simulink model "LQ_simulation"  (R2024b)
settings: Solver=VariableStepAuto  StartTime=0.0  StopTime=10.0  RelTol=1e-3
values from neighbouring files (symbols this model uses):
  A_kf = A_ext - L_kf*C_meas    [SS_model_LQ.m]
  A_x = [0, 1 ... (first row only)    [SS_model_LQ.m]
  B_kf = [L_kf B_ext]    [SS_model_LQ.m]
  B_x = [0; k2]    [SS_model_LQ.m]
  C_kf = eye(3)    [SS_model_LQ.m]
  C_x = [1, 0]    [SS_model_LQ.m]
  D_kf = zeros(3,3)    [SS_model_LQ.m]
  D_x = 0    [SS_model_LQ.m]
  K_lq = lqr(A_ext, B_ext, Q_lq, R_lq)    [SS_model_LQ.m]
  K_ref = -1/(C_pos_ext*((A_ext - B_ext*K_lq)\B_ext))    [SS_model_LQ.m]
  Kg = 3    [LQI_Giuse_code.m]    (also in SS_model_LQ.m)
  Ki_i = Ki_p/Ti    [LQI_Giuse_code.m]    (also in SS_model_LQ.m = 1650.02619)
  Kp_i = 72.795273    [SS_model_LQ.m]
  x_e = [x1_e, x2_e]    [LQI_Giuse_code.m]    (also in SS_model_LQ.m = 0.007)
undefined symbols (not defined in the file or in its folder): G_i_den, G_i_num
libraries: slpidlib x1
settings Model: Creator=edoardo  LastModifiedBy=edoardo

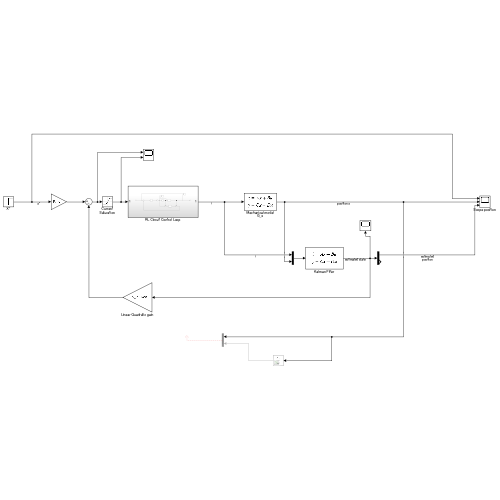
[thumbnail: Simulink's stored preview of the top-level diagram]
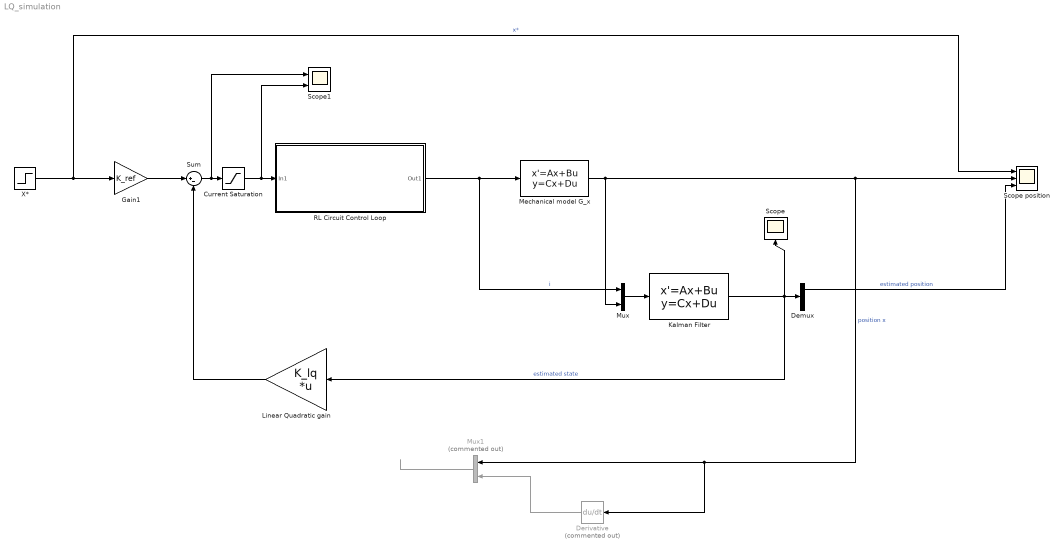
== system LQ_simulation ==
  Current Saturation : Saturate  UpperLimit=3  LowerLimit=-3
  Demux : Demux  Outputs=2
  Derivative : Derivative  Commented=on
  Gain1 : Gain  Gain=K_ref
  Kalman Filter : StateSpace  A=A_kf  B=B_kf  C=C_kf  D=D_kf  InitialCondition=0
  Linear Quadratic gain : Gain  Gain=K_lq  Multiplication=Matrix(K*u) (u vector)
  Mechanical model G_x : StateSpace  A=A_x  B=B_x  C=C_x  D=D_x  InitialCondition=0
  Mux : Mux  Inputs=2
  Mux1 : Mux  Commented=on  Inputs=2
  RL Circuit Control Loop : Subsystem
  Scope : Scope
  Scope position : Scope  NumInputPorts=3
  Scope1 : Scope  NumInputPorts=2
  Sum : Sum  Inputs=|+-
  X* : Step  After=x_e  SampleTime=0
  wires:
  RL Circuit Control Loop/1(Out1) -> Mux/1, Mechanical model G_x/1  "i"
  X*/1 -> Gain1/1, Scope position/1  "x*"
  Mechanical model G_x/1 -> Mux/2, Scope position/2, Mux1/1, Derivative/1  "position x"
  Mux/1 -> Kalman Filter/1
  Kalman Filter/1 -> Linear Quadratic gain/1, Scope/1, Demux/1  "estimated state"
  Linear Quadratic gain/1 -> Sum/2
  Sum/1 -> Scope1/1, Current Saturation/1
  Demux/1 -> Scope position/3  "estimated position"
  Current Saturation/1 -> Scope1/2, RL Circuit Control Loop/1(In1)
  Gain1/1 -> Sum/1
  Mux1/1 -> ?
  Derivative/1 -> Mux1/2

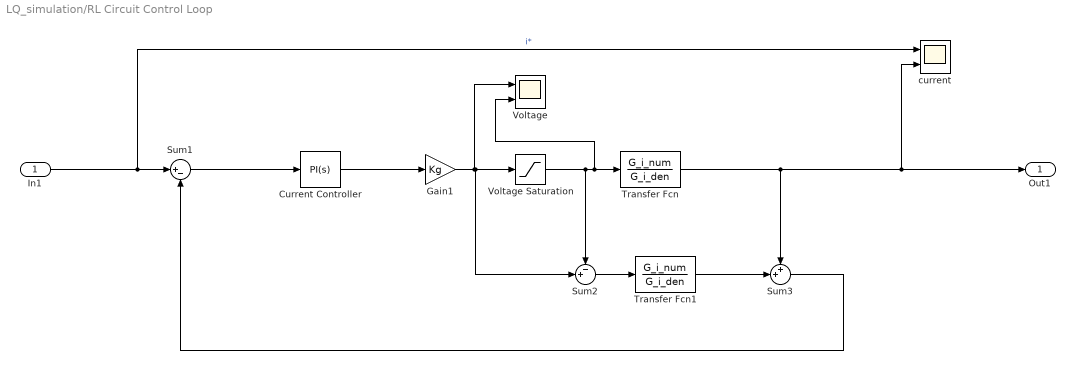
== system LQ_simulation/RL Circuit Control Loop ==
  In1 : Inport
  Current Controller : slpidlib/PID Controller  Controller=PI  Form=Parallel  TimeDomain=Continuous-time  UseExternalTs=off  SampleTime=-1  IntegratorMethod=Forward Euler  FilterMethod=Forward Euler  ControllerParametersSource=internal  P=Kp_i  I=Ki_i  UseKiTs=off  D=0  UseExternalDerivativeSource=off  N=100  UseFilter=on  TunerSelectOption=Transfer Function Based (PID Tuner App)  InitialConditionSource=internal  InitialConditionForIntegrator=0  InitialConditionForFilter=0  DifferentiatorICPrevScaledInput=0  ExternalReset=none  TrackingMode=off  Kt=1  LimitOutput=off  SatLimitsSource=internal  UpperSaturationLimit=inf  LowerSaturationLimit=-inf  LinearizeAsGain=on  AntiWindupMode=none  Kb=1  LimitIntegrator=off  UpperIntegratorSaturationLimit=inf  LowerIntegratorSaturationLimit=-inf  POutMin=[]  POutMax=[]  IOutMin=[]  IOutMax=[]  DOutMin=[]  DOutMax=[]  NOutMin=[]  NOutMax=[]  SumOutMin=[]  SumOutMax=[]  SaturationOutMin=[]  SaturationOutMax=[]  PParamMin=[]  PParamMax=[]  IParamMin=[]  IParamMax=[]  DParamMin=[]  DParamMax=[]  NParamMin=[]  NParamMax=[]  KbParamMin=[]  KbParamMax=[]  KtParamMin=[]  KtParamMax=[]  KbOutMin=[]  KbOutMax=[]  KtOutMin=[]  KtOutMax=[]  IntegratorOutMin=[]  IntegratorOutMax=[]  FilterOutMin=[]  FilterOutMax=[]  SumI1OutMin=[]  SumI1OutMax=[]  SumI2OutMin=[]  SumI2OutMax=[]  SumI3OutMin=[]  SumI3OutMax=[]  SumI4OutMin=[]  SumI4OutMax=[]  SumDOutMin=[]  SumDOutMax=[]  DifferentiatorOutMin=[]  DifferentiatorOutMax=[]  FilterDiffOutCoefMin=[]  FilterDiffOutCoefMax=[]  ReciprocalOutMin=[]  ReciprocalOutMax=[]  SumDenOutMin=[]  SumDenOutMax=[]  SumNumOutMin=[]  SumNumOutMax=[]  DivideOutMin=[]  DivideOutMax=[]  UdiffTsProdOutMin=[]  UdiffTsProdOutMax=[]  NTsProdOutMin=[]  NTsProdOutMax=[]  UintegralTsProdOutMin=[]  UintegralTsProdOutMax=[]  UngainTsProdOutMin=[]  UngainTsProdOutMax=[]  ClampingZeroOutDataTypeStr=Inherit: Inherit via back propagation  ClampingZeroOutMin=[]  ClampingZeroOutMax=[]  FilterDenConstantOutDataTypeStr=Inherit: Inherit via back propagation  FilterDenConstantOutMin=[]  FilterDenConstantOutMax=[]  PCopyOutDataTypeStr=Inherit: Inherit via back propagation  PCopyOutMin=[]  PCopyOutMax=[]  NCopyOutDataTypeStr=Inherit: Inherit via back propagation  NCopyOutMin=[]  NCopyOutMax=[]  IntegratorContinuousStateAttributes=''  IntegratorStateMustResolveToSignalObject=off  IntegratorRTWStateStorageClass=Auto  FilterContinuousStateAttributes=''  FilterStateMustResolveToSignalObject=off  FilterRTWStateStorageClass=Auto  ParallelPVariant=InternalParameters  IdealPVariant=Disabled  IVariant=InternalParameters  DVariant=Disabled  IntegratorVariant=Continuous  SatVariant=Disabled  AWVariant=Passthrough  PCopyVariant=Disabled  TRVariant=Disabled  FdbkBlocksVariant=Forward  IdealPFdbkVariant=Disabled  SatFdbkVariant=Disabled  DerivativeFilterVariant=Disabled  NVariant=Disabled  NCopyVariant=Disabled_SignalSpec  FilterICVariant=Disabled  IntegratorICVariant=InternalICs  ExternalResetVariant=Disabled  TRSumVariant=Passthrough  SumFdbkVariant=Disabled  SumVariant=Sum_PI  TsampFilterVariant=InternalTs  TsampNgainVariant=Passthrough  TsampIntegralVariant=Disabled_SignalSpec  ExternalSaturationOutDataTypeStr=Inherit: Same as second input  DerivativeSourceVariant=Disabled  PreIntVariant=InternalPreInt
  Gain1 : Gain  Gain=Kg
  Sum1 : Sum  Inputs=|+-
  Sum2 : Sum  Inputs=-+|
  Sum3 : Sum  Inputs=++|
  Transfer Fcn : TransferFcn  Numerator=G_i_num  Denominator=G_i_den
  Transfer Fcn1 : TransferFcn  Numerator=G_i_num  Denominator=G_i_den
  Voltage : Scope  NumInputPorts=2
  Voltage Saturation : Saturate  UpperLimit=24  LowerLimit=-24
  current : Scope  NumInputPorts=2
  Out1 : Outport
  wires:
  Sum1/1 -> Current Controller/1
  Sum2/1 -> Transfer Fcn1/1
  In1/1 -> current/1, Sum1/1  "i*"
  Voltage Saturation/1 -> Sum2/1, Voltage/2, Transfer Fcn/1
  Gain1/1 -> Sum2/2, Voltage Saturation/1, Voltage/1
  Transfer Fcn1/1 -> Sum3/2
  Sum3/1 -> Sum1/2
  Current Controller/1 -> Gain1/1
  Transfer Fcn/1 -> current/2, Out1/1, Sum3/1
